simulink model "Prey_Predator"  (R2017b)
settings: Solver=VariableStepAuto  StartTime=0.0  StopTime=10.0  RelTol=1e-3
InitFcn:
  | a=1
  | b=2
  | c=3
  | d=4
  | x1_0=d/c
  | x2_0=a/b
model workspace (MAT data in the model file):
  a = 1
  b = 2
  c = 3
  d = 4
settings Model: Creator=EloyR_5y442ym  LastModifiedBy=EloyR_5y442ym

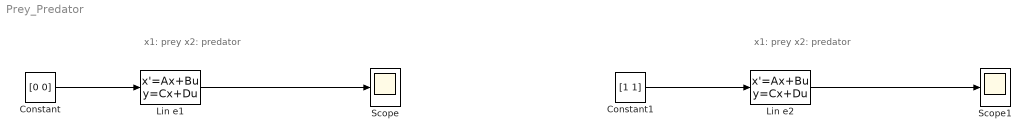
== system Prey_Predator ==
  note: x1: prey
      | x2: predator
  note: x1: prey
      | x2: predator
  Constant : Constant  Value=[0 0]
  Constant1 : Constant  Value=[1 1]
  Lin e1 : StateSpace  A=[a 0;0 -d]  B=[0 0;0 0]  C=[1 0; 0 1]  D=[0 0; 0 0]  InitialCondition=[x1_0; x2_0]  ContinuousStateAttributes='Lin.e1'
  Lin e2 : StateSpace  A=[0 -b*d/c; a*c/b 0]  B=[a*d/c 0; 0 -a*d/b]  C=[1 0; 0 1]  D=[0 0; 0 0]  InitialCondition=[x1_0; x2_0]  ContinuousStateAttributes='Lin.e2'
  Scope : Scope
  Scope1 : Scope
  wires:
  Constant/1 -> Lin e1/1
  Lin e1/1 -> Scope/1
  Lin e2/1 -> Scope1/1
  Constant1/1 -> Lin e2/1
